simulink subsystem "Subsystem_final"  (R2023b)
settings: Solver=VariableStepAuto  StartTime=0.0  StopTime=10.0  RelTol=1e-3
libraries: spsMosfetLib x2, spsOnDelayLib x2, spsSeriesRLCBranchLib x2, spsVoltageMeasurementLib x2, spsCurrentMeasurementLib x1, slpidlib x1
settings Model: Creator=zhaoxu  LastModifiedBy=zhaoxu

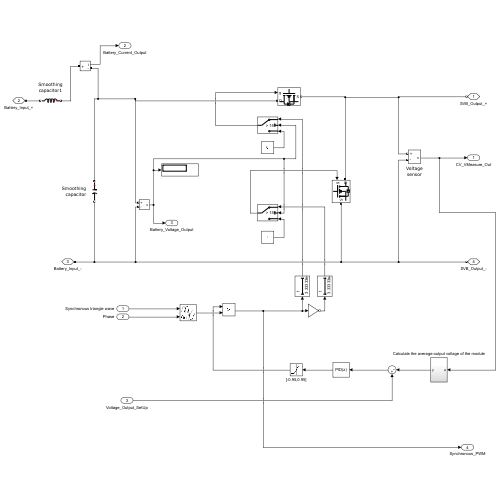
[thumbnail: Simulink's stored preview of the top-level diagram]
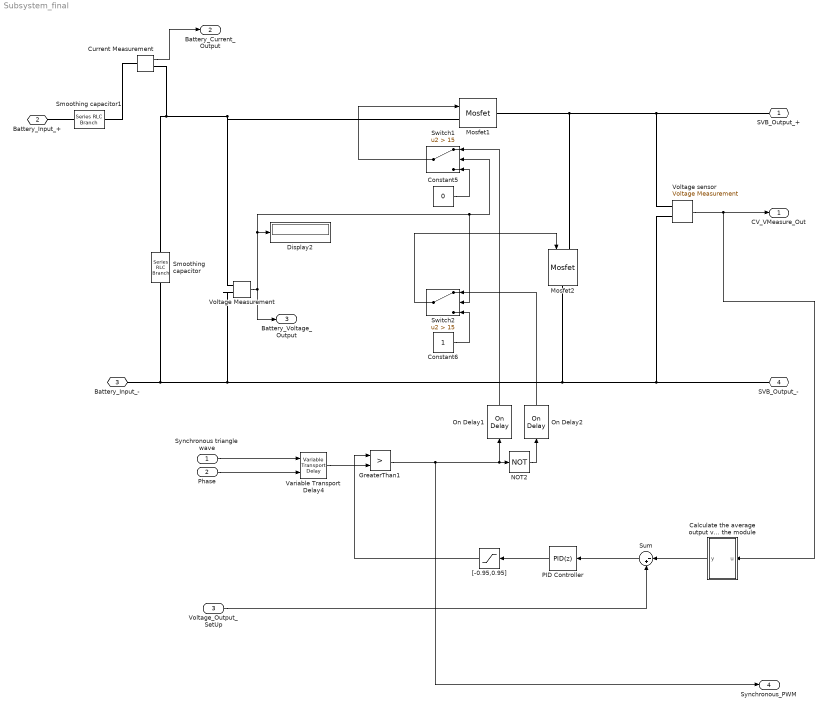
== system Subsystem_final ==
  Synchronous triangle wave : Inport
  Phase : Inport  Port=2
  Voltage_Output_SetUp : Inport  Port=3
  Calculate the average output voltage of the module : Subsystem
  Constant5 : Constant  Value=0
  Constant6 : Constant
  Current Measurement : spsCurrentMeasurementLib/Current Measurement  PhasorSimulation=off  OutputType=Complex  PSBequivalent=0
  Display2 : Display
  GreaterThan1 : RelationalOperator  Operator=>  OutDataTypeStr=boolean  RndMeth=Simplest  InputSameDT=off
  Mosfet1 : spsMosfetLib/Mosfet  Ron=1.7e-3  Lon=0  Rd=0.01  Vfd=0.9  IC=0  Rs=1e5  Cs=inf  Measurements=off
  Mosfet2 : spsMosfetLib/Mosfet  Ron=1.7e-3  Lon=0  Rd=0.01  Vfd=0.9  IC=0  Rs=1e5  Cs=inf  Measurements=off
  NOT2 : Logic  Operator=NOT  IconShape=distinctive  AllPortsSameDT=off  OutDataTypeStr=boolean
  On Delay1 : spsOnDelayLib/On Delay  DelayType=On delay  delay=1/5e4/60  ic=0  Ts=0
  On Delay2 : spsOnDelayLib/On Delay  DelayType=On delay  delay=1/5e4/60  ic=0  Ts=0
  PID Controller : slpidlib/PID Controller  Controller=PID  Form=Parallel  TimeDomain=Discrete-time  UseExternalTs=off  SampleTime=1e-4  IntegratorMethod=Forward Euler  FilterMethod=Forward Euler  ControllerParametersSource=internal  P=0.05  I=9  UseKiTs=off  D=0.0001  N=100  UseFilter=on  TunerSelectOption=Transfer Function Based (PID Tuner App)  InitialConditionSource=internal  InitialConditionForIntegrator=0  InitialConditionForFilter=0  DifferentiatorICPrevScaledInput=0  ExternalReset=none  TrackingMode=off  Kt=1  LimitOutput=off  SatLimitsSource=internal  UpperSaturationLimit=inf  LowerSaturationLimit=-inf  LinearizeAsGain=on  AntiWindupMode=none  Kb=1  LimitIntegrator=off  UpperIntegratorSaturationLimit=inf  LowerIntegratorSaturationLimit=-inf  POutMin=[]  POutMax=[]  IOutMin=[]  IOutMax=[]  DOutMin=[]  DOutMax=[]  NOutMin=[]  NOutMax=[]  SumOutMin=[]  SumOutMax=[]  SaturationOutMin=[]  SaturationOutMax=[]  PParamMin=[]  PParamMax=[]  IParamMin=[]  IParamMax=[]  DParamMin=[]  DParamMax=[]  NParamMin=[]  NParamMax=[]  KbParamMin=[]  KbParamMax=[]  KtParamMin=[]  KtParamMax=[]  KbOutMin=[]  KbOutMax=[]  KtOutMin=[]  KtOutMax=[]  IntegratorOutMin=[]  IntegratorOutMax=[]  FilterOutMin=[]  FilterOutMax=[]  SumI1OutMin=[]  SumI1OutMax=[]  SumI2OutMin=[]  SumI2OutMax=[]  SumI3OutMin=[]  SumI3OutMax=[]  SumI4OutMin=[]  SumI4OutMax=[]  SumDOutMin=[]  SumDOutMax=[]  DifferentiatorOutMin=[]  DifferentiatorOutMax=[]  FilterDiffOutCoefMin=[]  FilterDiffOutCoefMax=[]  ReciprocalOutMin=[]  ReciprocalOutMax=[]  SumDenOutMin=[]  SumDenOutMax=[]  SumNumOutMin=[]  SumNumOutMax=[]  DivideOutMin=[]  DivideOutMax=[]  UdiffTsProdOutMin=[]  UdiffTsProdOutMax=[]  NTsProdOutMin=[]  NTsProdOutMax=[]  UintegralTsProdOutMin=[]  UintegralTsProdOutMax=[]  UngainTsProdOutMin=[]  UngainTsProdOutMax=[]  ClampingZeroOutDataTypeStr=Inherit: Inherit via back propagation  ClampingZeroOutMin=[]  ClampingZeroOutMax=[]  FilterDenConstantOutDataTypeStr=Inherit: Inherit via back propagation  FilterDenConstantOutMin=[]  FilterDenConstantOutMax=[]  PCopyOutDataTypeStr=Inherit: Inherit via back propagation  PCopyOutMin=[]  PCopyOutMax=[]  NCopyOutDataTypeStr=Inherit: Inherit via back propagation  NCopyOutMin=[]  NCopyOutMax=[]  IntegratorContinuousStateAttributes=''  IntegratorStateMustResolveToSignalObject=off  IntegratorRTWStateStorageClass=Auto  FilterContinuousStateAttributes=''  FilterStateMustResolveToSignalObject=off  FilterRTWStateStorageClass=Auto  ParallelPVariant=InternalParameters  IdealPVariant=Disabled  IVariant=InternalParameters  DVariant=InternalParameters  IntegratorVariant=Discrete  SatVariant=Disabled  AWVariant=Passthrough  PCopyVariant=Disabled  TRVariant=Disabled  FdbkBlocksVariant=Forward  IdealPFdbkVariant=Disabled  SatFdbkVariant=Disabled  DerivativeFilterVariant=ForwardEulerFilter  NVariant=InternalParameters  NCopyVariant=Disabled  FilterICVariant=InternalICsFilter  IntegratorICVariant=InternalICs  ExternalResetVariant=Disabled  TRSumVariant=Passthrough  SumFdbkVariant=Disabled  SumVariant=Sum_PID  TsampFilterVariant=InternalTs  TsampNgainVariant=Passthrough  TsampIntegralVariant=Disabled_SignalSpec  ExternalSaturationOutDataTypeStr=Inherit: Same as second input
  Smoothing capacitor : spsSeriesRLCBranchLib/Series RLC Branch  LConnTagsString=__new0  RConnTagsString=__new0  BranchType=C  Resistance=1  Inductance=1e-3  SetiL0=off  InitialCurrent=0  Capacitance=7.22e-5  Setx0=off  InitialVoltage=0  Measurements=None
  Smoothing capacitor1 : spsSeriesRLCBranchLib/Series RLC Branch  LConnTagsString=__new0  RConnTagsString=__new0  BranchType=L  Resistance=1  Inductance=5e-7  SetiL0=off  InitialCurrent=0  Capacitance=7.22e-5  Setx0=off  InitialVoltage=0  Measurements=None
  Sum : Sum  Inputs=|-+  InputSameDT=on  SaturateOnIntegerOverflow=on  OutDataTypeStr=Inherit: Same as first input
  Switch1 : Switch  Criteria=u2 > Threshold  Threshold=15  SaturateOnIntegerOverflow=off  InputSameDT=off
  Switch2 : Switch  Criteria=u2 > Threshold  Threshold=15  SaturateOnIntegerOverflow=off  InputSameDT=off
  Variable Transport Delay4 : VariableTransportDelay  MaximumDelay=10
  Voltage sensor : spsVoltageMeasurementLib/Voltage Measurement  PhasorSimulation=off  OutputType=Complex  PSBequivalent=0
  Voltage Measurement : spsVoltageMeasurementLib/Voltage Measurement  PhasorSimulation=off  OutputType=Complex  PSBequivalent=0
  "[-0.95,0.95]" : Saturate  UpperLimit=0.95  LowerLimit=-0.95
  SVB_Output_+ : PMIOPort  Side=Right
  Battery_Input_+ : PMIOPort  Port=2  Side=Left
  Battery_Input_- : PMIOPort  Port=3  Side=Left
  SVB_Output_- : PMIOPort  Port=4  Side=Right
  CV_VMeasure_Out : Outport
  Battery_Current_Output : Outport  Port=2
  Battery_Voltage_Output : Outport  Port=3
  Synchronous_PWM : Outport  Port=4
  wires:
  Current Measurement/1 -> Battery_Current_Output/1
  NOT2/1 -> On Delay2/1
  GreaterThan1/1 -> NOT2/1, On Delay1/1, Synchronous_PWM/1
  Phase/1 -> Variable Transport Delay4/2
  Synchronous triangle wave/1 -> Variable Transport Delay4/1
  Constant5/1 -> Switch1/3
  Switch1/1 -> Mosfet1/1
  Constant6/1 -> Switch2/3
  Switch2/1 -> Mosfet2/1
  Voltage Measurement/1 -> Battery_Voltage_Output/1, Display2/1, Switch2/2, Switch1/2
  Voltage_Output_SetUp/1 -> Sum/2
  Variable Transport Delay4/1 -> GreaterThan1/2
  PID Controller/1 -> "[-0.95,0.95]"/1
  Sum/1 -> PID Controller/1
  On Delay1/1 -> Switch1/1
  On Delay2/1 -> Switch2/1
  "[-0.95,0.95]"/1 -> GreaterThan1/1
  Voltage sensor/1 -> CV_VMeasure_Out/1, Calculate the average output voltage of the module/1(u)
  Calculate the average output voltage of the module/1(y) -> Sum/1
  connections:
  Mosfet1/LConn1 -- Current Measurement/RConn1 -- Smoothing capacitor/LConn1 -- Voltage Measurement/LConn1
  Battery_Input_-/RConn1 -- SVB_Output_-/RConn1 -- Voltage sensor/LConn2 -- Mosfet2/RConn1 -- Voltage Measurement/LConn2 -- Smoothing capacitor/RConn1
  Voltage sensor/LConn1 -- Mosfet1/RConn1 -- Mosfet2/LConn1 -- SVB_Output_+/RConn1
  Smoothing capacitor1/RConn1 -- Battery_Input_+/RConn1
  Smoothing capacitor1/LConn1 -- Current Measurement/LConn1

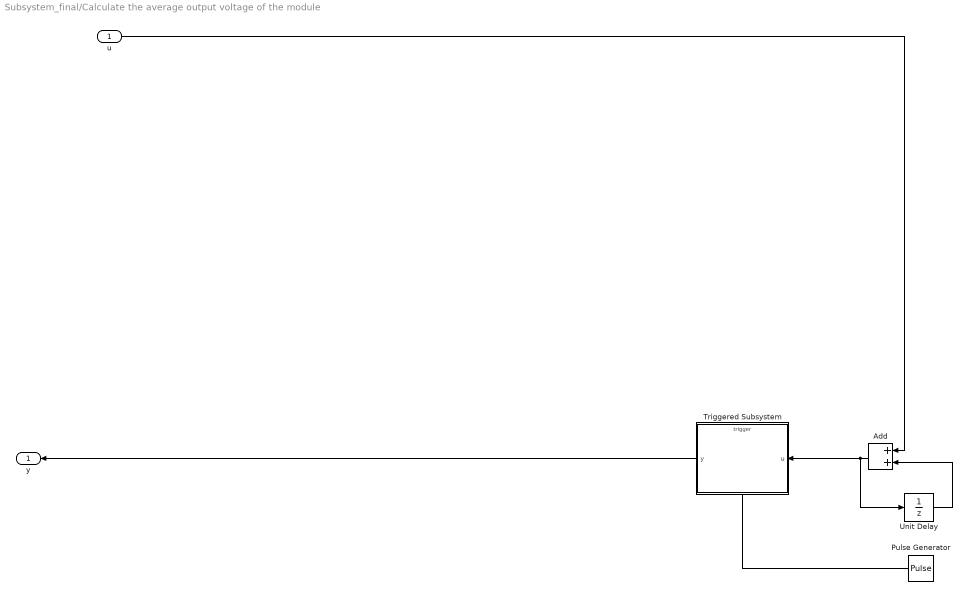
== system Subsystem_final/Calculate the average output voltage of the module ==
  u : Inport
  Add : Sum
  Pulse Generator : DiscretePulseGenerator  PulseType=Time based  Period=1e-4  PulseWidth=50
  Triggered Subsystem : Subsystem  TreatAsAtomicUnit=on
  Unit Delay : UnitDelay  SampleTime=1/5e4/60  HasFrameUpgradeWarning=on
  y : Outport
  wires:
  u/1 -> Add/1
  Triggered Subsystem/1(y) -> y/1
  Unit Delay/1 -> Add/2
  Pulse Generator/1 -> Triggered Subsystem/Trigger
  Add/1 -> Triggered Subsystem/1(u), Unit Delay/1

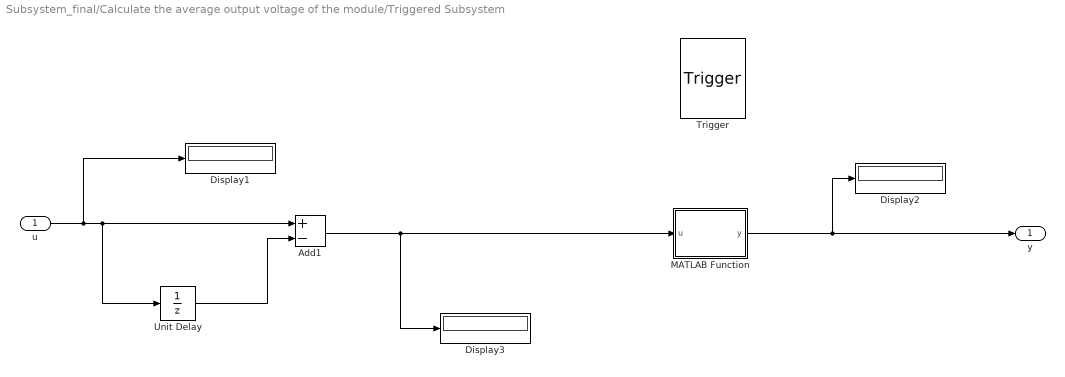
== system Subsystem_final/Calculate the average output voltage of the module/Triggered Subsystem ==
  u : Inport
  Trigger : TriggerPort  VariantControl=(inherit)
  Add1 : Sum  Inputs=+-
  Display1 : Display
  Display2 : Display
  Display3 : Display
  MATLAB Function : MATLAB Function  TreatAsAtomicUnit=on
  Unit Delay : UnitDelay  SampleTime=-1  HasFrameUpgradeWarning=on
  y : Outport
  wires:
  Unit Delay/1 -> Add1/2
  Add1/1 -> MATLAB Function/1(u), Display3/1
  u/1 -> Add1/1, Unit Delay/1, Display1/1
  MATLAB Function/1(y) -> y/1, Display2/1

== matlab function Subsystem_final/Calculate the average output voltage of the module/Triggered Subsystem/MATLAB Function ==
  data: u input; y output
function y = fcn(u)
%#codegen

y = u / 300;
